simulink model "pendulum_nonlinear"  (Simulink 8.5)
settings: Solver=ode23t  StartTime=0.0  StopTime=T  RelTol=1e-3
InitFcn:
  | T=1000;
  | seed1=now()*rand(1,1);
  | seed2=now()*rand(1,1);
  | seed3=now()*rand(1,1);
  | seed4=now()*rand(1,1);
settings Model: Creator=tjohnson  LastModifiedBy=tjohnson
settings DataIOCC: SignalLoggingSaveFormat=Dataset
settings OptimizationCC: ExpressionDepthLimit=128
settings DebuggingCC: UnderspecifiedInitializationDetection=Simplified  MergeDetectMultiDrivingBlocksExec=error  FcnCallInpInsideContextMsg=EnableAllAsError  StateNameClashWarn=none
settings GRTTargetCC: CombineOutputUpdateFcns=on  GRTInterface=off

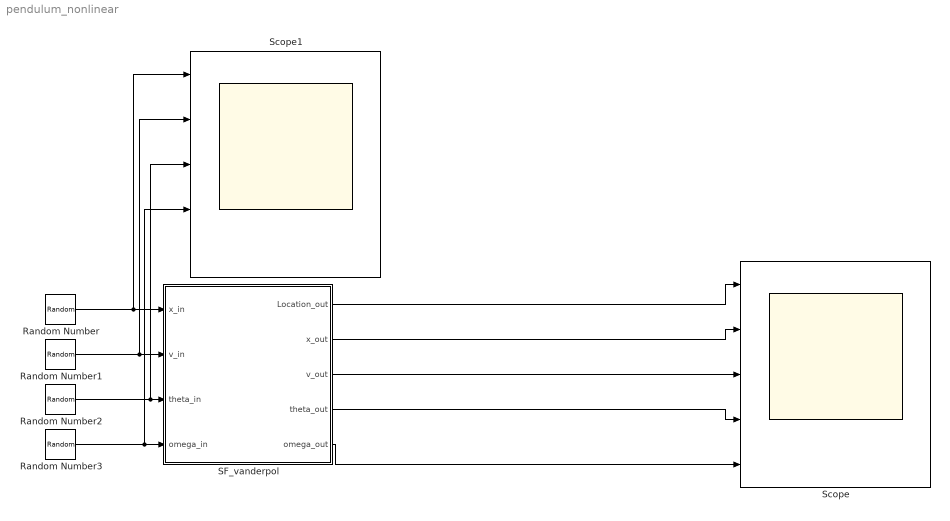
== system pendulum_nonlinear ==
  Random Number : RandomNumber  Variance=5  Seed=seed1  SampleTime=T
  Random Number1 : RandomNumber  Variance=5  Seed=seed2  SampleTime=T
  Random Number2 : RandomNumber  Variance=5  Seed=seed3  SampleTime=T
  Random Number3 : RandomNumber  Variance=5  Seed=seed4  SampleTime=T
  SF_vanderpol : Stateflow chart  TreatAsAtomicUnit=on
  Scope : Scope  NumInputPorts=5
      settings: YMin=0~-700~0~1.568~1  YMax=1.2e+10~700~6.5e+10~1.5735~1  DataFormat=Structure
  Scope1 : Scope  NumInputPorts=5
      settings: YMin=0~-700~0~1.568~0.95  YMax=1.2e+10~700~6.5e+10~1.5735~1.05  DataFormat=Structure
  wires:
  SF_vanderpol/2(x_out) -> Scope/2
  SF_vanderpol/5(omega_out) -> Scope/5
  SF_vanderpol/1(Location_out) -> Scope/1
  SF_vanderpol/3(v_out) -> Scope/3
  SF_vanderpol/4(theta_out) -> Scope/4
  Random Number/1 -> Scope1/1, SF_vanderpol/1(x_in)
  Random Number3/1 -> Scope1/4, SF_vanderpol/4(omega_in)
  Random Number2/1 -> Scope1/3, SF_vanderpol/3(theta_in)
  Random Number1/1 -> Scope1/2, SF_vanderpol/2(v_in)

== stateflow chart SF_vanderpol ==
  settings: updateMethod=CONTINUOUS
  state running
    du:
    x_dot = v;
    v_dot = -(omega^2*sin(theta) - (5401*v)/1900 + cos(theta)*((3*omega)/2500 + (147*sin(theta))/5))/(3*cos(theta)^2 - 29);
    theta_dot = omega;
    omega_dot = ((87*omega)/2500 + (4263*sin(theta))/5 - cos(theta)*(- 3*sin(theta)*omega^2 + (16203*v)/1900))/(3*cos(theta)^2 - 29);
    x_out=x;
    v_out=v;
    theta_out=theta;
    omega_out=omega;
    Location_out =1;
  running -> running [order 2] : [theta <= -2*pi]
      | {theta=0;}
  running -> running [order 1] : [theta >= 2*pi]
      | {theta=0;}
  (default) -> running : {x = x_in; v = v_in; theta=theta_in; omega=omega_in;}
  data: Location_out output double; x local double; x_out output double; omega local double; v local double; v_out output double; theta_out output double; omega_out output double; theta local double; x_in input double; v_in input double; theta_in input double; omega_in input double
  data x settings: updateMethod=SF_CONTINUOUS_TIME_DATA
  data omega settings: updateMethod=SF_CONTINUOUS_TIME_DATA
  data v settings: updateMethod=SF_CONTINUOUS_TIME_DATA
  data theta settings: updateMethod=SF_CONTINUOUS_TIME_DATA
  data x_in settings: updateMethod=SF_CONTINUOUS_TIME_DATA
  data v_in settings: updateMethod=SF_CONTINUOUS_TIME_DATA
  data theta_in settings: updateMethod=SF_CONTINUOUS_TIME_DATA
  data omega_in settings: updateMethod=SF_CONTINUOUS_TIME_DATA
